simulink model "FIR_InterpolationFilter_Ex1"  (R2025a)
settings: Solver=VariableStepAuto  StartTime=0.0  StopTime=0.2  RelTol=1e-3
PostLoadFcn:
  | % All frequency values are in Hz.
  | Fs = 250000;  % Sampling Frequency
  | Fpass = 19000;            % Passband Frequency
  | Fstop = 31000;            % Stopband Frequency
  | Dpass = 0.00460513763;    % Passband Ripple
  | Dstop = 0.0001;           % Stopband Attenuation
  | dens  = 16;               % Density Factor
  | % Calculate the order from the parameters using FIRPMORD.
  | [N, Fo, Ao, W] = firpmord([Fpass, Fstop]/(Fs/2), [1 0], [Dpass, Dstop]);
  | % Calculate the coefficients using the FIRPM function.
  | b  = firpm(N, Fo, Ao, W, {dens});
  | coeffs = b;
undefined symbols (not defined in the file): None, S, vsva2197, xcvc1902
libraries: aieDSP x1, dspsrcs4 x1, dspmlti4 x1, vmcUtilities x1
settings Model: Creator=robg  LastModifiedBy=robg
settings DebuggingCC: ParameterPrecisionLossMsg=none  UnconnectedInputMsg=warning  UnconnectedOutputMsg=warning  UnconnectedLineMsg=warning
settings ModelReferenceCC: EnableRefExpFcnMdlSchedulingChecks=on
settings RTWCC: GPUComputeCapability=3.5  DLArmComputeVersion=19.05

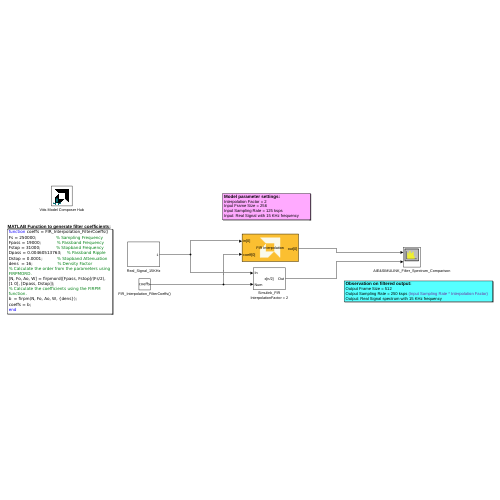
[thumbnail: Simulink's stored preview of the top-level diagram]
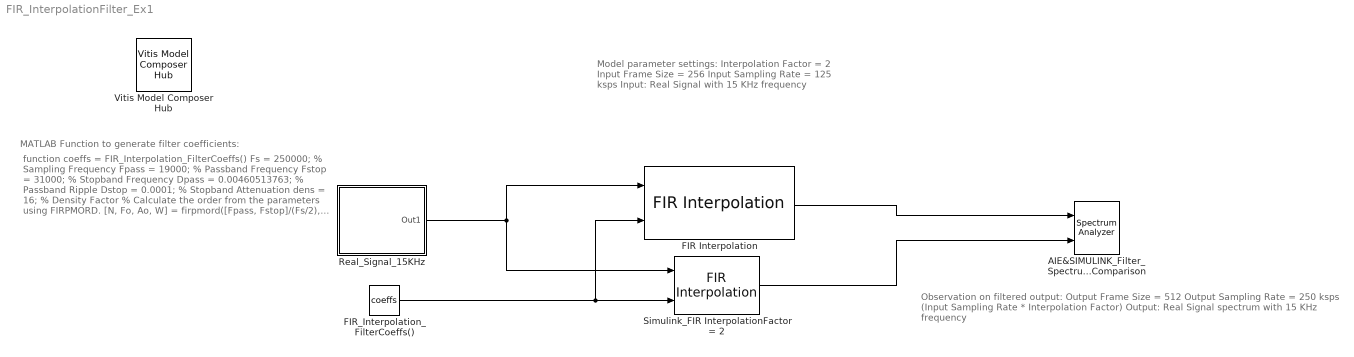
== system FIR_InterpolationFilter_Ex1 ==
  note: MATLAB Function to generate filter coefficients:
  note: function coeffs = FIR_Interpolation_FilterCoeffs()
      | Fs = 250000; % Sampling Frequency
      | Fpass = 19000; % Passband Frequency
      | Fstop = 31000; % Stopband Frequency
      | Dpass = 0.00460513763; % Passband Ripple
      | Dstop = 0.0001; % Stopband Attenuation
      | dens = 16; % Density Factor
      | % Calculate the order from the parameters using FIRPMORD.
      | [N, Fo, Ao, W] = firpmord([Fpass, Fstop]/(Fs/2), [1 0], [Dpass, Dstop]);
      | % Calculate the coefficients using the FIRPM function.
      | b = firpm(N, Fo, Ao, W, {dens});
      | coeffs = b;
      | end
  note: Model parameter settings:
      | Interpolation Factor = 2
      | Input Frame Size = 256
      | Input Sampling Rate = 125 ksps
      | Input: Real Signal with 15 KHz frequency
  note: Observation on filtered output:
      | Output Frame Size = 512
      | Output Sampling Rate = 250 ksps (Input Sampling Rate * Interpolation Factor)
      | Output: Real Signal spectrum with 15 KHz frequency
  AIE&SIMULINK_Filter_Spectrum_Comparison : SpectrumAnalyzer  NumInputPorts=2  AveragingMethod=Exponential  ShowLegend=on  ChannelNames="[\"\"]"  AllowFFTLengthLessThanSamplesPerUpdate=on  DefaultConfigurationName=spbscopes.SpectrumAnalyzerBlockCfg
  FIR Interpolation : aieDSP/FIR Interpolation  data_type=float  coef_type=float  use_coeff_reload=on  num_outputs=off  coeff=[1, zeros(1,31)]  fir_length=72  interpolate_factor=2  input_window_size=256  shift_val=0  rnd_mode=Round to positive infinity  sat_mode=0-None  interp_poly=1  casc_length=1  AIE_VARIANT=1  TP_API=0  dual_ip=0  ssr=1  blockJsonConstraints=[]  blockJsonConstraintsInternal=[]  spec=vmc_fir_interpolate_asym.json  SerializedMaskParamNames=[]  SerializedMaskParamValues=[]  SerializedMaskParamVisibilities=[]  block_type=FIR Interpolation  SerializedMaskParamDataypes=typename|typename|uint|uint|coef_type|uint|uint|uint|uint|uint|uint|uint|uint|uint|uint|uint|uint  SerializedMaskParamEnumStrArr=0|0|0|0|0|0|0|0|0|Floor,Ceiling,Round to positive infinity,Round to negative infinity,Round symmetrical to infinity,Round symmetrical to zero,Round convergent to even,Round convergent to odd|0-None,1-Asymmetric,3-Symmetric|0|0|0|0|0|0  SerializedMaskParamEnumValArr=0|0|0|0|0|0|0|0|0|0,1,2,3,4,5,6,7|0,1,3|0|0|0|0|0|0  SerializedMaskParamVectorArr=0|0|0|0|1|0|0|0|0|0|0|0|0|0|0|0|0  SerializedMaskParamKeys=TT_DATA|TT_COEFF|TP_USE_COEFF_RELOAD|TP_NUM_OUTPUTS|coeff|TP_FIR_LEN|TP_INTERPOLATE_FACTOR|TP_INPUT_WINDOW_VSIZE|TP_SHIFT|TP_RND|TP_SAT|TP_PARA_INTERP_POLY|TP_CASC_LEN|AIE_VARIANT|TP_API|TP_DUAL_IP|TP_SSR
  FIR_Interpolation_FilterCoeffs() : Constant  Value=coeffs  OutDataTypeStr=single
  Real_Signal_15KHz : Subsystem
  Simulink_FIR InterpolationFactor = 2 : dspmlti4/FIR Interpolation  FilterSource=Input port  PrivateCoeffs=0  h=coeffs  L=2  FilterObject=FINTERP  InputProcessing=Columns as channels (frame based)  framing=Enforce single-rate processing  outputBufInitCond=0  roundingMode=Ceiling  overflowMode=off  firstCoeffDataTypeStr=Inherit: Same word length as input  firstCoeffMin=[]  firstCoeffMax=[]  firstCoeffLastDataTypeStr=Inherit: Same word length as input  outputMin=[]  outputMax=[]
  Vitis Model Composer Hub : vmcUtilities/Vitis Model Composer Hub  Tag=genX  CodeGeneration=off  StartColumn=1  NumberOfColumns=1  TargetDirectory=./code  exportDesign=off  analyzeDesign=off  validateDesignOnHw=off  ExportType=AI Engines  IpVendor=xilinx.com  IpLibrary=hls  IpVersion=1.0  IpHWLanguage=Verilog  AieCompilerOptions={}  AieSimulatorOptions={}  CreateTestbench=off  TestbenchStackSize=10  RunRtlSim=off  RunCSim=off  RunAieSim=off  enableSimulationTimeout=on  enableGraphIterations=on  AieSimTimeout=50000  AieGraphIterations=-1  RunAieSimProfiling=off  LaunchVitisAnalyzer=off  PlotOutput=off  RunX86Sim=off  X86SimTimeout=10  GenHwImage=off  GenLibadfXo=off  GenHwValidationCode=off  PlatformType=Not Specified  HwSystemType=Baremetal  HwValidationTarget=hw  ProjDevice=xcvc1902-vsva2197-1LP-e-S  ProjDevicePart=xcvc1902-vsva2197-1LP-e-S  AIEType=AIE  SamplePeriod=-1  ClockFrequency=200  DataPathParallelism=1  xilinxfamily=versalaicore  part=xcvc1902  speed=-1LP-e-S  package=vsva2197  directory=./netlist  testbench=off  incr_netlist=off  synthesis_tool=Vivado  clock_wrapper=Clock Enables  dbl_ovrd=According to Block Masks  dcm_input_clock_period=10  sysclk_period=10  simulink_period=1  eval_field=0  LogFileName=''  NThreads=4
  wires:
  Real_Signal_15KHz/1(Out1) -> FIR Interpolation/1, Simulink_FIR InterpolationFactor = 2/1
  FIR_Interpolation_FilterCoeffs()/1 -> FIR Interpolation/2, Simulink_FIR InterpolationFactor = 2/2
  FIR Interpolation/1 -> AIE&SIMULINK_Filter_Spectrum_Comparison/1
  Simulink_FIR InterpolationFactor = 2/1 -> AIE&SIMULINK_Filter_Spectrum_Comparison/2

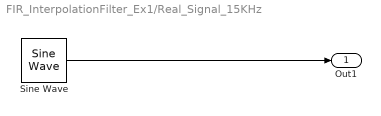
== system FIR_InterpolationFilter_Ex1/Real_Signal_15KHz ==
  Sine Wave : dspsrcs4/Sine Wave  Amplitude=1  Frequency=15e3  Phase=0  SampleMode=Discrete  OutComplex=Real  CompMethod=Trigonometric fcn  TableSize=Speed  SampleTime=1/125e3  SamplesPerFrame=256  ResetState=Restart at time zero  OutputFrames=off  dataType=single  wordLen=16  udDataType=sfix(16)  fracBitsMode=Best precision  numFracBits=15  OutDataTypeStr=single  LastOutDataTypeStr=single
  Out1 : Outport
  wires:
  Sine Wave/1 -> Out1/1
